simulink library "find6DoFSBFGS_cl"  (R2018b)
settings: Solver=VariableStepAuto  StartTime=0.0  StopTime=10.0  RelTol=1e-3
values from neighbouring files (symbols this model uses):
  botCamPositionVec_cm = reshape(botCamPositionVec_cm,[3,1])    [find6DoFSBFGS_init.m]
  GFC2Bottom = calculateRotationMatrix(botEulerAngles_rad(1),botEulerAngles_rad(2),botEulerAngles_rad(3))    [find6DoFSBFGS_init.m]
  GFC2Side = calculateRotationMatrix(sideEulerAngles_rad(1),sideEulerAngles_rad(2),sideEulerAngles_rad(3))    [find6DoFSBFGS_init.m]
  GFC2Slant = calculateRotationMatrix(slantEulerAngles_rad(1),slantEulerAngles_rad(2),slantEulerAngles_rad(3))    [find6DoFSBFGS_init.m]
  sideCamPositionVec_cm = reshape(sideCamPositionVec_cm,[3,1])    [find6DoFSBFGS_init.m]
  slantCamPositionVec_cm = reshape(slantCamPositionVec_cm,[3,1])    [find6DoFSBFGS_init.m]
libraries: FindUnitVectorComponents_ul x4, rayTrace_ul x4, findEulerAngles_ul x1, findUnitVectors_ul x1, snellLeastSquaresPosition_ul x1
settings Model: Creator=mcobb  LastModifiedBy=M.Cobb

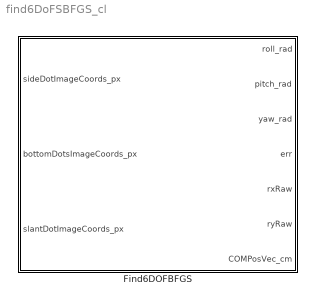
== system find6DoFSBFGS_cl ==
  Find6DOFBFGS : Subsystem  mask{Parameter1=0}
      mask Callback Parameter1: setCamNumClbk
      mask Display:
      | image('find6DoFSBFGSBlockImage.png',[.2, .2, .6, .6],'on');
      | 
      | % port_label('input',1,'Side')
      | % port_label('input',2,'Bottom')
      | % port_label('input',3,'Back')
      | 
      | port_label('output',1,'eulAngVec_rad')
      | port_label('output',2,'CoMPosVec_cm')
      | port_label('output',3,'err')
      | 
      | text(0.5, 1, 'BFGS - Resolve 6 DOF', 'horizontalAlignment', 'center', ...
      |   'verticalAlignment', 'top')

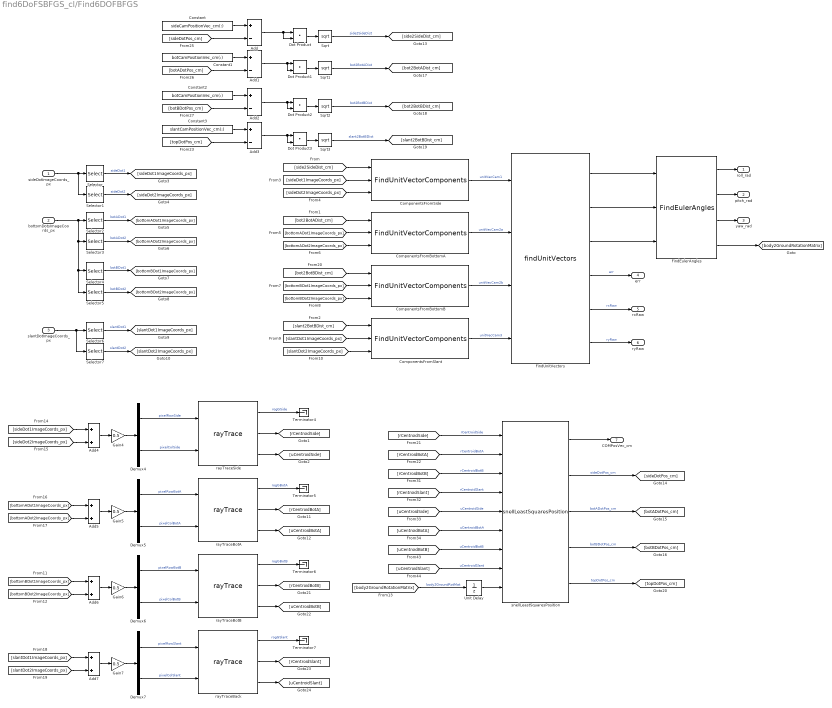
== system find6DoFSBFGS_cl/Find6DOFBFGS ==
  sideDotImageCoords_px : Inport
  bottomDotsImageCoords_px : Inport  Port=2
  slantDotImageCoords_px : Inport  Port=3
  Add{,1..3} (4 alike) : Sum  Inputs=+-
  Add{4..7} (4 alike) : Sum
  ComponentsFromBottomA : FindUnitVectorComponents_ul/FindUnitVectorComponents  cameraViewAngleVec_deg=cameraFOVAngles_deg  cam2GroundRotationMatrix=GFC2Bottom'  imageDimensions=imageDims_px
  ComponentsFromBottomB : FindUnitVectorComponents_ul/FindUnitVectorComponents  cameraViewAngleVec_deg=cameraFOVAngles_deg  cam2GroundRotationMatrix=GFC2Bottom'  imageDimensions=imageDims_px
  ComponentsFromSide : FindUnitVectorComponents_ul/FindUnitVectorComponents  cameraViewAngleVec_deg=cameraFOVAngles_deg  cam2GroundRotationMatrix=GFC2Side'  imageDimensions=imageDims_px
  ComponentsFromSlant : FindUnitVectorComponents_ul/FindUnitVectorComponents  cameraViewAngleVec_deg=cameraFOVAngles_deg  cam2GroundRotationMatrix=GFC2Slant'  imageDimensions=imageDims_px
  Constant : Constant  Value=sideCamPositionVec_cm(:)
  Constant1 : Constant  Value=botCamPositionVec_cm(:)
  Constant2 : Constant  Value=botCamPositionVec_cm(:)
  Constant3 : Constant  Value=slantCamPositionVec_cm(:)
  Demux{4..7} (4 alike) : Demux  Outputs=2
  Dot Product{,1..3} (4 alike) : DotProduct  InputSameDT=on  OutDataTypeStr=Inherit: Inherit via internal rule
  FindEulerAngles : findEulerAngles_ul/FindEulerAngles  SystemSampleTime=-1
  FindUnitVectors : findUnitVectors_ul/findUnitVectors  sideSeparation_cm=sideSeparation_cm  bottomASeparation_cm=bottomASeparation_cm  bottomBSeparation_cm=bottomBSeparation_cm  topSeparation_cm=topSeparation_cm  DSB=DSB  DBL=DBL
  Gain{4..7} (4 alike) : Gain  Gain=0.5
  Selector : Selector  InputPortWidth=4  IndexOptions=Index vector (dialog)  Indices=[1 2]  OutputSizes=1
  Selector1 : Selector  InputPortWidth=4  IndexOptions=Index vector (dialog)  Indices=[3 4]  OutputSizes=1
  Selector2 : Selector  InputPortWidth=8  IndexOptions=Index vector (dialog)  Indices=[1 2]  OutputSizes=1
  Selector3 : Selector  InputPortWidth=8  IndexOptions=Index vector (dialog)  Indices=[3 4]  OutputSizes=1
  Selector4 : Selector  InputPortWidth=8  IndexOptions=Index vector (dialog)  Indices=[5 6]  OutputSizes=1
  Selector5 : Selector  InputPortWidth=8  IndexOptions=Index vector (dialog)  Indices=[7 8]  OutputSizes=1
  Selector6 : Selector  InputPortWidth=4  IndexOptions=Index vector (dialog)  Indices=[1 2]  OutputSizes=1
  Selector7 : Selector  InputPortWidth=4  IndexOptions=Index vector (dialog)  Indices=[3 4]  OutputSizes=1
  Sqrt{,1..3} (4 alike) : Sqrt  SaturateOnIntegerOverflow=on
  Terminator{4..7} (4 alike) : Terminator
  Unit Delay : UnitDelay  InitialCondition=eye(3)  SampleTime=-1
  rayTraceBack : rayTrace_ul/rayTrace  camPosVec_cm=slantCamPositionVec_cm  camEulAngles_deg=slantEulerAngles_deg  dist2Glass_cm=slantCamDistToGlass_cm  indOfRefVec=indxOfRefVec  glassPlane=3  glassThickness_cm=prscGlassThick_cm  imageDimsVec_px=imageDims_px  camFOV_deg=cameraFOVAngles_deg  Periscope=1
  rayTraceBotA : rayTrace_ul/rayTrace  camPosVec_cm=botCamPositionVec_cm  camEulAngles_deg=botEulerAngles_deg  dist2Glass_cm=botCamDistToGlass_cm  indOfRefVec=indxOfRefVec  glassPlane=1  glassThickness_cm=glassThickness_cm  imageDimsVec_px=imageDims_px  camFOV_deg=cameraFOVAngles_deg  Periscope=1
  rayTraceBotB : rayTrace_ul/rayTrace  camPosVec_cm=botCamPositionVec_cm  camEulAngles_deg=botEulerAngles_deg  dist2Glass_cm=botCamDistToGlass_cm  indOfRefVec=indxOfRefVec  glassPlane=1  glassThickness_cm=glassThickness_cm  imageDimsVec_px=imageDims_px  camFOV_deg=cameraFOVAngles_deg  Periscope=1
  rayTraceSide : rayTrace_ul/rayTrace  camPosVec_cm=sideCamPositionVec_cm  camEulAngles_deg=sideEulerAngles_deg  dist2Glass_cm=sideCamDistToGlass_cm  indOfRefVec=indxOfRefVec  glassPlane=2  glassThickness_cm=glassThickness_cm  imageDimsVec_px=imageDims_px  camFOV_deg=cameraFOVAngles_deg  Periscope=1
  snellLeastSquaresPosition : snellLeastSquaresPosition_ul/snellLeastSquaresPosition  sideDotPosVec_cm=sidePositionVecBF_cm  botADotPosVec_cm=botAPositionVecBF_cm  botBDotPosVec_cm=botBPositionVecBF_cm  topDotPosVec_cm=topPositionVecBF_cm
  roll_rad : Outport  Unit=rad
  pitch_rad : Outport  Port=2  Unit=rad
  yaw_rad : Outport  Port=3  Unit=rad
  err : Outport  Port=4
  rxRaw : Outport  Port=5
  ryRaw : Outport  Port=6
  COMPosVec_cm : Outport  Port=7  Unit=rad
  wires:
  ComponentsFromSide/1 -> FindUnitVectors/1  "unitVecCam1"
  ComponentsFromBottomA/1 -> FindUnitVectors/2  "unitVecCam2a"
  ComponentsFromBottomB/1 -> FindUnitVectors/3  "unitVecCam2b"
  ComponentsFromSlant/1 -> FindUnitVectors/4  "unitVecCam3"
  FindUnitVectors/2 -> FindEulerAngles/2
  FindUnitVectors/1 -> FindEulerAngles/1
  FindUnitVectors/3 -> FindEulerAngles/3
  [sideDot1ImageCoords_px] -> ComponentsFromSide/2
  [sideDot2ImageCoords_px] -> ComponentsFromSide/3
  [bottomADot1ImageCoords_px] -> ComponentsFromBottomA/2
  [bottomADot2ImageCoords_px] -> ComponentsFromBottomA/3
  [bottomBDot1ImageCoords_px] -> ComponentsFromBottomB/2
  [bottomBDot2ImageCoords_px] -> ComponentsFromBottomB/3
  [slantDot1ImageCoords_px] -> ComponentsFromSlant/2
  [slantDot2ImageCoords_px] -> ComponentsFromSlant/3
  FindEulerAngles/1 -> roll_rad/1
  FindEulerAngles/2 -> pitch_rad/1
  FindEulerAngles/3 -> yaw_rad/1
  FindUnitVectors/4 -> err/1  "err"
  [side2SideDist_cm] -> ComponentsFromSide/1
  [bot2BotADist_cm] -> ComponentsFromBottomA/1
  [slant2BotBDist_cm] -> ComponentsFromSlant/1
  [bot2BotBDist_cm] -> ComponentsFromBottomB/1
  Selector/1 -> [sideDot1ImageCoords_px]  "sideDot1"
  Selector1/1 -> [sideDot2ImageCoords_px]  "sideDot2"
  sideDotImageCoords_px/1 -> Selector1/1, Selector/1
  bottomDotsImageCoords_px/1 -> Selector5/1, Selector4/1, Selector3/1, Selector2/1
  Selector2/1 -> [bottomADot1ImageCoords_px]  "botADot1"
  Selector3/1 -> [bottomADot2ImageCoords_px]  "botADot2"
  Selector4/1 -> [bottomBDot1ImageCoords_px]  "botBDot1"
  Selector5/1 -> [bottomBDot2ImageCoords_px]  "botBDot2"
  Selector6/1 -> [slantDot1ImageCoords_px]  "slantDot1"
  slantDotImageCoords_px/1 -> Selector7/1, Selector6/1
  Selector7/1 -> [slantDot2ImageCoords_px]  "slantDot2"
  FindUnitVectors/5 -> rxRaw/1  "rxRaw"
  FindUnitVectors/6 -> ryRaw/1  "ryRaw"
  FindEulerAngles/4 -> [body2GroundRotationMatrix]
  rayTraceBotA/3 -> [uCentroidBotA]
  Demux6/2 -> rayTraceBotB/2  "pixelColBotB"
  rayTraceBotB/1 -> Terminator6/1  "rogGBotB"
  Demux6/1 -> rayTraceBotB/1  "pixelRowBotB"
  Gain6/1 -> Demux6/1
  Gain7/1 -> Demux7/1
  rayTraceBotA/1 -> Terminator5/1  "rogGBotA"
  Add7/1 -> Gain7/1
  rayTraceBotB/2 -> [rCentroidBotB]
  Add4/1 -> Gain4/1
  [sideDot1ImageCoords_px] -> Add4/1
  rayTraceSide/3 -> [uCentroidSide]
  [bottomADot1ImageCoords_px] -> Add5/1
  Add6/1 -> Gain6/1
  Add5/1 -> Gain5/1
  Gain5/1 -> Demux5/1
  Gain4/1 -> Demux4/1
  Demux5/1 -> rayTraceBotA/1  "pixelRowBotA"
  rayTraceSide/1 -> Terminator4/1  "rogGSide"
  Demux4/1 -> rayTraceSide/1  "pixelRowSide"
  [slantDot2ImageCoords_px] -> Add7/2
  rayTraceBack/3 -> [uCentroidSlant]
  Demux7/1 -> rayTraceBack/1  "pixelRowSlant"
  [uCentroidBotA] -> snellLeastSquaresPosition/6  "uCentroidBotA"
  rayTraceBack/1 -> Terminator7/1  "rogGSlant"
  [sideDot2ImageCoords_px] -> Add4/2
  Demux7/2 -> rayTraceBack/2  "pixelColSlant"
  [bottomADot2ImageCoords_px] -> Add5/2
  [slantDot1ImageCoords_px] -> Add7/1
  [bottomBDot2ImageCoords_px] -> Add6/2
  rayTraceBack/2 -> [rCentroidSlant]
  [uCentroidSlant] -> snellLeastSquaresPosition/8  "uCentroidSlant"
  Demux4/2 -> rayTraceSide/2  "pixelColSide"
  rayTraceSide/2 -> [rCentroidSide]
  [bottomBDot1ImageCoords_px] -> Add6/1
  [uCentroidBotB] -> snellLeastSquaresPosition/7  "uCentroidBotB"
  rayTraceBotA/2 -> [rCentroidBotA]
  [rCentroidSlant] -> snellLeastSquaresPosition/4  "rCentroidSlant"
  [rCentroidBotA] -> snellLeastSquaresPosition/2  "rCentroidBotA"
  [rCentroidSide] -> snellLeastSquaresPosition/1  "rCentroidSide"
  [body2GroundRotationMatrix] -> Unit Delay/1  "body2GroundRotMat"
  [rCentroidBotB] -> snellLeastSquaresPosition/3  "rCentroidBotB"
  rayTraceBotB/3 -> [uCentroidBotB]
  [uCentroidSide] -> snellLeastSquaresPosition/5  "uCentroidSide"
  Demux5/2 -> rayTraceBotA/2  "pixelColBotA"
  snellLeastSquaresPosition/1 -> COMPosVec_cm/1
  snellLeastSquaresPosition/2 -> [sideDotPos_cm]  "sideDotPos_cm"
  snellLeastSquaresPosition/3 -> [botADotPos_cm]  "botADotPos_cm"
  snellLeastSquaresPosition/4 -> [botBDotPos_cm]  "botBDotPos_cm"
  Constant/1 -> Add/1
  [sideDotPos_cm] -> Add/2
  Add/1 -> Dot Product/1, Dot Product/2
  Sqrt/1 -> [side2SideDist_cm]  "side2SideDist"
  Add1/1 -> Dot Product1/2, Dot Product1/1
  Add2/1 -> Dot Product2/2, Dot Product2/1
  Add3/1 -> Dot Product3/2, Dot Product3/1
  Sqrt1/1 -> [bot2BotADist_cm]  "bot2BotADist"
  Sqrt2/1 -> [bot2BotBDist_cm]  "bot2BotBDist"
  Sqrt3/1 -> [slant2BotBDist_cm]  "slant2BotBDist"
  [botADotPos_cm] -> Add1/2
  [botBDotPos_cm] -> Add2/2
  [topDotPos_cm] -> Add3/2
  Constant1/1 -> Add1/1
  Constant2/1 -> Add2/1
  Constant3/1 -> Add3/1
  Dot Product/1 -> Sqrt/1
  Dot Product1/1 -> Sqrt1/1
  Dot Product2/1 -> Sqrt2/1
  Dot Product3/1 -> Sqrt3/1
  Unit Delay/1 -> snellLeastSquaresPosition/9
  snellLeastSquaresPosition/5 -> [topDotPos_cm]  "topDotPos_cm"
